simulink model "c2000_host_CAN_acceptance_filtering"  (R2021b)
settings: Solver=VariableStepAuto  StartTime=0.0  StopTime=Inf  RelTol=1e-3  EnableMultiTasking=on
undefined symbols (not defined in the file or in its folder): canChannel
libraries: canlib x9, canmsglib x8, demo_controls x1
settings Model: ExtModeTrigDuration=8  Creator=The MathWorks, Inc.  LastModifiedBy=The MathWorks, Inc.
settings SolverCC: AlgebraicLoopSolver=TrustRegion
settings DebuggingCC: SFMachineParentedDataDiag=warning

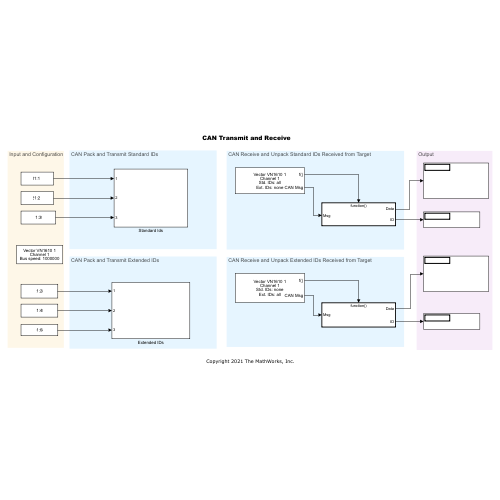
[thumbnail: Simulink's stored preview of the top-level diagram]
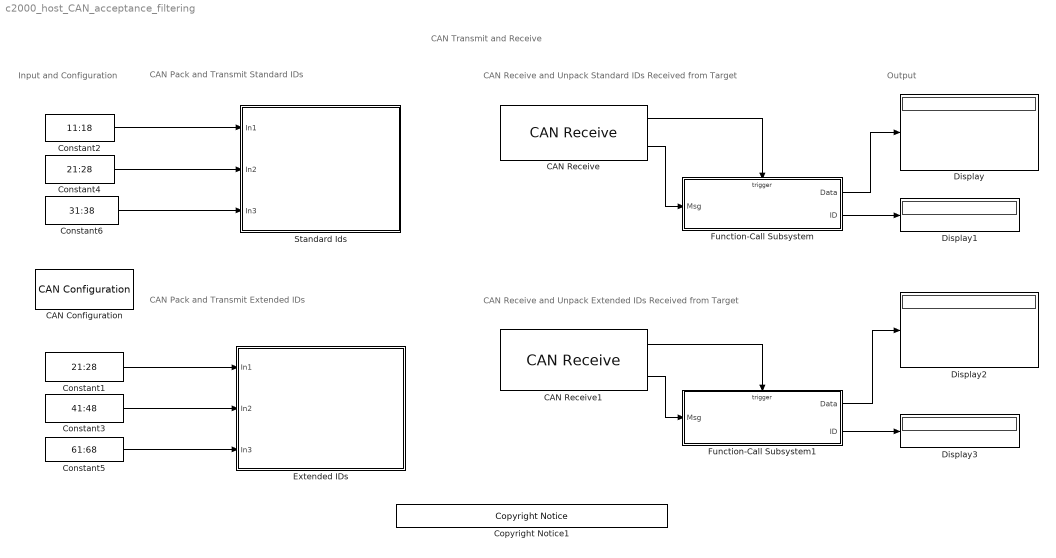
== system c2000_host_CAN_acceptance_filtering ==
  note: CAN Transmit and Receive
  note: Input and Configuration
  note: CAN Pack and Transmit Standard IDs
  note: CAN Pack and Transmit Extended IDs
  note: Output
  note: CAN Receive and Unpack Standard IDs Received from Target
  note: CAN Receive and Unpack Extended IDs Received from Target
  CAN Configuration : canlib/CAN Configuration  BlockHandle=2.0149  Device=MathWorks Virtual 1 (Channel 1)  DeviceMenu=MathWorks Virtual 1 (Channel 1)  ObjConstructor=canChannel('MathWorks', 'Virtual 1', 1)  BusSpeed=1000000  EnableBitParameters=off  SJW=1  TSEG1=4  TSEG2=3  NSamples=1  AckMode=Normal
      settings: SourceProductBaseCode=VN
  CAN Receive : canlib/CAN Receive  Priority=40  BlockHandle=3.0149  Device=MathWorks Virtual 1 (Channel 1)  DeviceMenu=MathWorks Virtual 1 (Channel 1)  ObjConstructor=canChannel('MathWorks', 'Virtual 1', 1)  EnableStandardIDsFilter=off  StdIDsCombo=Allow all  StandardIDs=0  EnableExtendedIDsFilter=off  ExtIDsCombo=Block all  ExtendedIDs=hex2dec('0x0000C000')  SampleTime=0.001  MsgsPerTimestep=1  InternalFilterUpdateStatus=on  BusOutput=off
      settings: SourceProductBaseCode=VN
  CAN Receive1 : canlib/CAN Receive  Priority=40  BlockHandle=4.0149  Device=MathWorks Virtual 1 (Channel 1)  DeviceMenu=MathWorks Virtual 1 (Channel 1)  ObjConstructor=canChannel('MathWorks', 'Virtual 1', 1)  EnableStandardIDsFilter=off  StdIDsCombo=Block all  StandardIDs=0  EnableExtendedIDsFilter=off  ExtIDsCombo=Allow all  ExtendedIDs=hex2dec('0x0000C000')  SampleTime=0.001  MsgsPerTimestep=all  InternalFilterUpdateStatus=on  BusOutput=off
      settings: SourceProductBaseCode=VN
  Constant1 : Constant  Value=21:28  OutDataTypeStr=uint8  SampleTime=0.005
  Constant2 : Constant  Value=11:18  OutDataTypeStr=uint8  SampleTime=0.005
  Constant3 : Constant  Value=41:48  OutDataTypeStr=uint8  SampleTime=0.007
  Constant4 : Constant  Value=21:28  OutDataTypeStr=uint8  SampleTime=0.007
  Constant5 : Constant  Value=61:68  OutDataTypeStr=uint8  SampleTime=0.009
  Constant6 : Constant  Value=31:38  OutDataTypeStr=uint8  SampleTime=0.009
  Copyright Notice1 : demo_controls/Copyright Notice  year=2021  prod=tic2000
      settings: SourceProductBaseCode=ME
  Display{,1..3} (4 alike) : Display
      Display1 settings: Format=hex (Stored Integer)
      Display3 settings: Format=hex (Stored Integer)
  Extended IDs : Subsystem
  Function-Call Subsystem : Subsystem  TreatAsAtomicUnit=on
  Function-Call Subsystem1 : Subsystem  TreatAsAtomicUnit=on
  Standard Ids : Subsystem  Priority=30
  wires:
  Constant2/1 -> Standard Ids/1(In1)
  Constant4/1 -> Standard Ids/2(In2)
  Constant6/1 -> Standard Ids/3(In3)
  CAN Receive/2 -> Function-Call Subsystem/1(Msg)
  CAN Receive/1 -> Function-Call Subsystem/Trigger
  Function-Call Subsystem/1(Data) -> Display/1
  Function-Call Subsystem/2(ID) -> Display1/1
  Constant1/1 -> Extended IDs/1(In1)
  Constant3/1 -> Extended IDs/2(In2)
  Constant5/1 -> Extended IDs/3(In3)
  Function-Call Subsystem1/2(ID) -> Display3/1
  CAN Receive1/2 -> Function-Call Subsystem1/1(Msg)
  Function-Call Subsystem1/1(Data) -> Display2/1
  CAN Receive1/1 -> Function-Call Subsystem1/Trigger

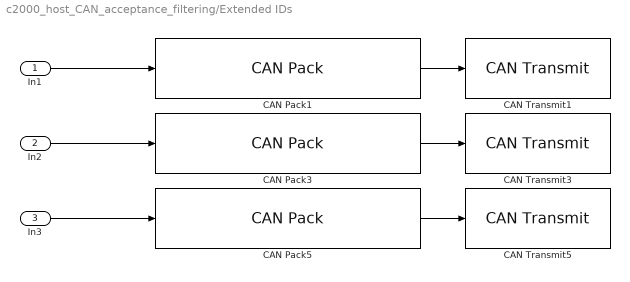
== system c2000_host_CAN_acceptance_filtering/Extended IDs ==
  In1 : Inport
  In2 : Inport  Port=2
  In3 : Inport  Port=3
  CAN Pack1 : canmsglib/CAN Pack  MsgList=(none)  MsgName=CAN Msg  MsgIDType=Extended (29-bit identifier)  MsgIdentifier=hex2dec('0x1C00000B')  MsgLength=8  Remote=off  ApplyMinMax=off  BusOutput=off  SignalInfo={}
      settings: SourceProductBaseCode=ME,XP,VN  DataFormat=raw data
  CAN Pack3 : canmsglib/CAN Pack  MsgList=(none)  MsgName=CAN Msg  MsgIDType=Extended (29-bit identifier)  MsgIdentifier=hex2dec('0x1C000003')  MsgLength=8  Remote=off  ApplyMinMax=off  BusOutput=off  SignalInfo={}
      settings: SourceProductBaseCode=ME,XP,VN  DataFormat=raw data
  CAN Pack5 : canmsglib/CAN Pack  MsgList=(none)  MsgName=CAN Msg  MsgIDType=Extended (29-bit identifier)  MsgIdentifier=hex2dec('0x1C000007')  MsgLength=8  Remote=off  ApplyMinMax=off  BusOutput=off  SignalInfo={}
      settings: SourceProductBaseCode=ME,XP,VN  DataFormat=raw data
  CAN Transmit1 : canlib/CAN Transmit  BlockHandle=23.0165  Device=MathWorks Virtual 1 (Channel 1)  DeviceMenu=MathWorks Virtual 1 (Channel 1)  ObjConstructor=canChannel('MathWorks', 'Virtual 1', 1)  EnableEventTransmit=off  EnablePeriodicTransmit=on  MessagePeriod=0.005
      settings: SourceProductBaseCode=VN
  CAN Transmit3 : canlib/CAN Transmit  BlockHandle=24.0161  Device=MathWorks Virtual 1 (Channel 1)  DeviceMenu=MathWorks Virtual 1 (Channel 1)  ObjConstructor=canChannel('MathWorks', 'Virtual 1', 1)  EnableEventTransmit=off  EnablePeriodicTransmit=on  MessagePeriod=0.007
      settings: SourceProductBaseCode=VN
  CAN Transmit5 : canlib/CAN Transmit  BlockHandle=25.0159  Device=MathWorks Virtual 1 (Channel 1)  DeviceMenu=MathWorks Virtual 1 (Channel 1)  ObjConstructor=canChannel('MathWorks', 'Virtual 1', 1)  EnableEventTransmit=off  EnablePeriodicTransmit=on  MessagePeriod=0.009
      settings: SourceProductBaseCode=VN
  wires:
  CAN Pack5/1 -> CAN Transmit5/1
  CAN Pack1/1 -> CAN Transmit1/1
  CAN Pack3/1 -> CAN Transmit3/1
  In1/1 -> CAN Pack1/1
  In2/1 -> CAN Pack3/1
  In3/1 -> CAN Pack5/1

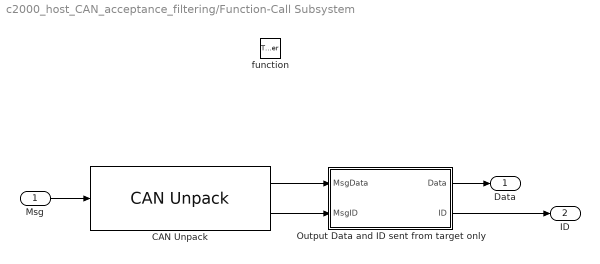
== system c2000_host_CAN_acceptance_filtering/Function-Call Subsystem ==
  Msg : Inport
  function : TriggerPort  TriggerType=function-call  VariantControl=(inherit)
  CAN Unpack : canmsglib/CAN Unpack  MsgList=(none)  MsgName=CAN Msg  MsgIDType=Extended (29-bit identifier)  MsgIdentifier=-1  MsgLength=8  SignalInfo={}  IDPort=on  TimestampPort=off  ErrorPort=off  RemotePort=off  LengthPort=off  StatusPort=off  ApplyMinMax=off
      settings: SourceProductBaseCode=ME,XP,VN  DataFormat=raw data
  "Output Data and ID sent from target only " : Subsystem
  Data : Outport
  ID : Outport  Port=2
  wires:
  Msg/1 -> CAN Unpack/1
  CAN Unpack/1 -> "Output Data and ID sent from target only "/1(MsgData)
  CAN Unpack/2 -> "Output Data and ID sent from target only "/2(MsgID)
  "Output Data and ID sent from target only "/1(Data) -> Data/1
  "Output Data and ID sent from target only "/2(ID) -> ID/1

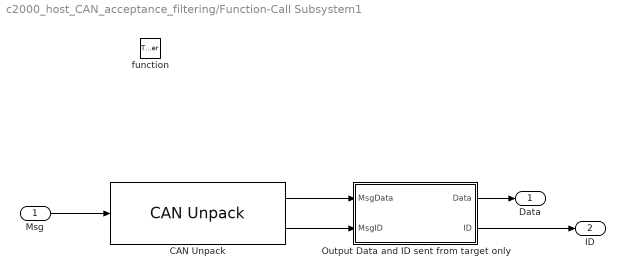
== system c2000_host_CAN_acceptance_filtering/Function-Call Subsystem1 ==
  Msg : Inport
  function : TriggerPort  TriggerType=function-call  VariantControl=(inherit)
  CAN Unpack : canmsglib/CAN Unpack  MsgList=(none)  MsgName=CAN Msg  MsgIDType=Extended (29-bit identifier)  MsgIdentifier=-1  MsgLength=8  SignalInfo={}  IDPort=on  TimestampPort=off  ErrorPort=off  RemotePort=off  LengthPort=off  StatusPort=off  ApplyMinMax=off
      settings: SourceProductBaseCode=ME,XP,VN  DataFormat=raw data
  "Output Data and ID sent from target only " : Subsystem
  Data : Outport
  ID : Outport  Port=2
  wires:
  Msg/1 -> CAN Unpack/1
  CAN Unpack/1 -> "Output Data and ID sent from target only "/1(MsgData)
  CAN Unpack/2 -> "Output Data and ID sent from target only "/2(MsgID)
  "Output Data and ID sent from target only "/1(Data) -> Data/1
  "Output Data and ID sent from target only "/2(ID) -> ID/1

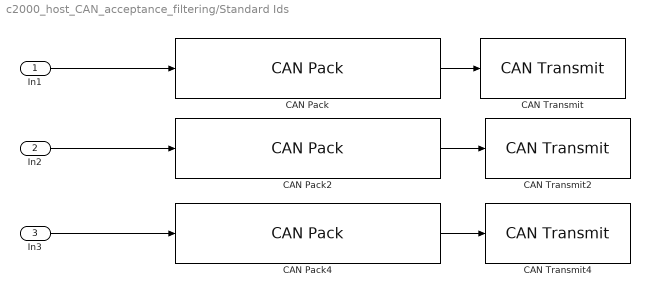
== system c2000_host_CAN_acceptance_filtering/Standard Ids ==
  In1 : Inport
  In2 : Inport  Port=2
  In3 : Inport  Port=3
  CAN Pack : canmsglib/CAN Pack  MsgList=(none)  MsgName=CAN Msg  MsgIDType=Standard (11-bit identifier)  MsgIdentifier=hex2dec('0x00000371')  MsgLength=8  Remote=off  ApplyMinMax=off  BusOutput=off  SignalInfo={}
      settings: SourceProductBaseCode=ME,XP,VN  DataFormat=raw data
  CAN Pack2 : canmsglib/CAN Pack  MsgList=(none)  MsgName=CAN Msg  MsgIDType=Standard (11-bit identifier)  MsgIdentifier=hex2dec('0x00000372')  MsgLength=8  Remote=off  ApplyMinMax=off  BusOutput=off  SignalInfo={}
      settings: SourceProductBaseCode=ME,XP,VN  DataFormat=raw data
  CAN Pack4 : canmsglib/CAN Pack  MsgList=(none)  MsgName=CAN Msg  MsgIDType=Standard (11-bit identifier)  MsgIdentifier=hex2dec('0x00000374')  MsgLength=8  Remote=off  ApplyMinMax=off  BusOutput=off  SignalInfo={}
      settings: SourceProductBaseCode=ME,XP,VN  DataFormat=raw data
  CAN Transmit : canlib/CAN Transmit  BlockHandle=200.01  Device=MathWorks Virtual 1 (Channel 1)  DeviceMenu=MathWorks Virtual 1 (Channel 1)  ObjConstructor=canChannel('MathWorks', 'Virtual 1', 1)  EnableEventTransmit=off  EnablePeriodicTransmit=on  MessagePeriod=0.005
      settings: SourceProductBaseCode=VN
  CAN Transmit2 : canlib/CAN Transmit  BlockHandle=201.0103  Device=MathWorks Virtual 1 (Channel 1)  DeviceMenu=MathWorks Virtual 1 (Channel 1)  ObjConstructor=canChannel('MathWorks', 'Virtual 1', 1)  EnableEventTransmit=off  EnablePeriodicTransmit=on  MessagePeriod=0.007
      settings: SourceProductBaseCode=VN
  CAN Transmit4 : canlib/CAN Transmit  BlockHandle=202.0106  Device=MathWorks Virtual 1 (Channel 1)  DeviceMenu=MathWorks Virtual 1 (Channel 1)  ObjConstructor=canChannel('MathWorks', 'Virtual 1', 1)  EnableEventTransmit=off  EnablePeriodicTransmit=on  MessagePeriod=0.009
      settings: SourceProductBaseCode=VN
  wires:
  In2/1 -> CAN Pack2/1
  In1/1 -> CAN Pack/1
  CAN Pack2/1 -> CAN Transmit2/1
  CAN Pack/1 -> CAN Transmit/1
  CAN Pack4/1 -> CAN Transmit4/1
  In3/1 -> CAN Pack4/1

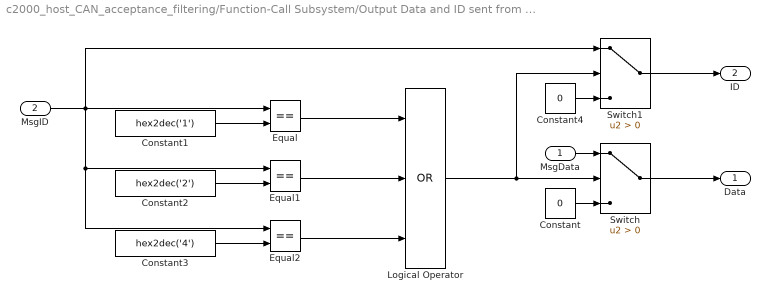
== system c2000_host_CAN_acceptance_filtering/Function-Call Subsystem/Output Data and ID sent from target only  ==
  MsgData : Inport
  MsgID : Inport  Port=2
  Constant : Constant  Value=0
  Constant1 : Constant  Value=hex2dec('1')
  Constant2 : Constant  Value=hex2dec('2')
  Constant3 : Constant  Value=hex2dec('4')
  Constant4 : Constant  Value=0
  Equal : RelationalOperator  Operator===  OutDataTypeStr=boolean  RndMeth=Simplest
  Equal1 : RelationalOperator  Operator===  OutDataTypeStr=boolean  RndMeth=Simplest
  Equal2 : RelationalOperator  Operator===  OutDataTypeStr=boolean  RndMeth=Simplest
  Logical Operator : Logic  Operator=OR  Inputs=3  AllPortsSameDT=off  OutDataTypeStr=boolean
  Switch : Switch  Criteria=u2 > Threshold  OutDataTypeStr=uint8
  Switch1 : Switch  Criteria=u2 > Threshold  OutDataTypeStr=uint32
  Data : Outport
  ID : Outport  Port=2
  wires:
  Constant/1 -> Switch/3
  Constant1/1 -> Equal/2
  Equal/1 -> Logical Operator/1
  MsgID/1 -> Switch1/1, Equal2/1, Equal1/1, Equal/1
  Equal2/1 -> Logical Operator/3
  Switch/1 -> Data/1
  Constant2/1 -> Equal1/2
  Equal1/1 -> Logical Operator/2
  Constant3/1 -> Equal2/2
  MsgData/1 -> Switch/1
  Logical Operator/1 -> Switch1/2, Switch/2
  Switch1/1 -> ID/1
  Constant4/1 -> Switch1/3

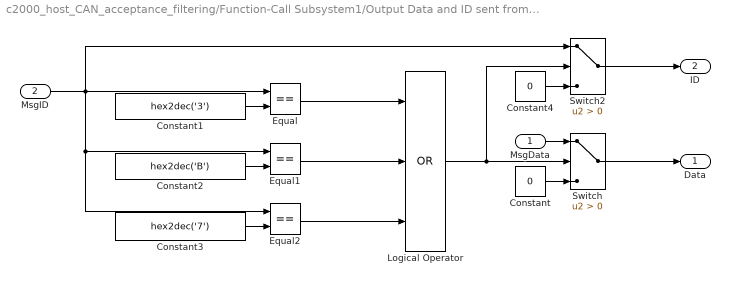
== system c2000_host_CAN_acceptance_filtering/Function-Call Subsystem1/Output Data and ID sent from target only  ==
  MsgData : Inport
  MsgID : Inport  Port=2
  Constant : Constant  Value=0
  Constant1 : Constant  Value=hex2dec('3')
  Constant2 : Constant  Value=hex2dec('B')
  Constant3 : Constant  Value=hex2dec('7')
  Constant4 : Constant  Value=0
  Equal : RelationalOperator  Operator===  OutDataTypeStr=boolean  RndMeth=Simplest
  Equal1 : RelationalOperator  Operator===  OutDataTypeStr=boolean  RndMeth=Simplest
  Equal2 : RelationalOperator  Operator===  OutDataTypeStr=boolean  RndMeth=Simplest
  Logical Operator : Logic  Operator=OR  Inputs=3  AllPortsSameDT=off  OutDataTypeStr=boolean
  Switch : Switch  Criteria=u2 > Threshold  OutDataTypeStr=uint8
  Switch2 : Switch  Criteria=u2 > Threshold  OutDataTypeStr=uint8
  Data : Outport
  ID : Outport  Port=2
  wires:
  Constant/1 -> Switch/3
  Constant1/1 -> Equal/2
  Equal/1 -> Logical Operator/1
  MsgID/1 -> Equal2/1, Equal1/1, Switch2/1, Equal/1
  Equal2/1 -> Logical Operator/3
  Switch/1 -> Data/1
  Constant2/1 -> Equal1/2
  Equal1/1 -> Logical Operator/2
  Constant3/1 -> Equal2/2
  MsgData/1 -> Switch/1
  Logical Operator/1 -> Switch2/2, Switch/2
  Switch2/1 -> ID/1
  Constant4/1 -> Switch2/3
